simulink model "PMSM_Motor"  (R2013b)
settings: Solver=ode45  StartTime=0.0  StopTime=1  MaxStep=1e-4  RelTol=1e-3
values from neighbouring files (symbols this model uses):
  B = 0    [PMSM_Motorsimulator.m]
  f = 60    [PMSM_Motorsimulator.m]
  J = 0.0001584    [PMSM_Motorsimulator.m]
  L_d = 5.7e-3    (= 0.0057)    [PMSM_Motorsimulator.m]
  L_q = 12.5e-3    (= 0.0125)    [PMSM_Motorsimulator.m]
  Phi_pm = 175e-3    (= 0.175)    [PMSM_Motorsimulator.m]
  Rs = 1.2    [PMSM_Motorsimulator.m]
  T_Load = 10    [PMSM_Motorsimulator.m]
  U = 230    [PMSM_Motorsimulator.m]
  Zp = 2    [PMSM_Motorsimulator.m]
settings Model: Creator=ahakimi  LastModifiedBy=ahakimi

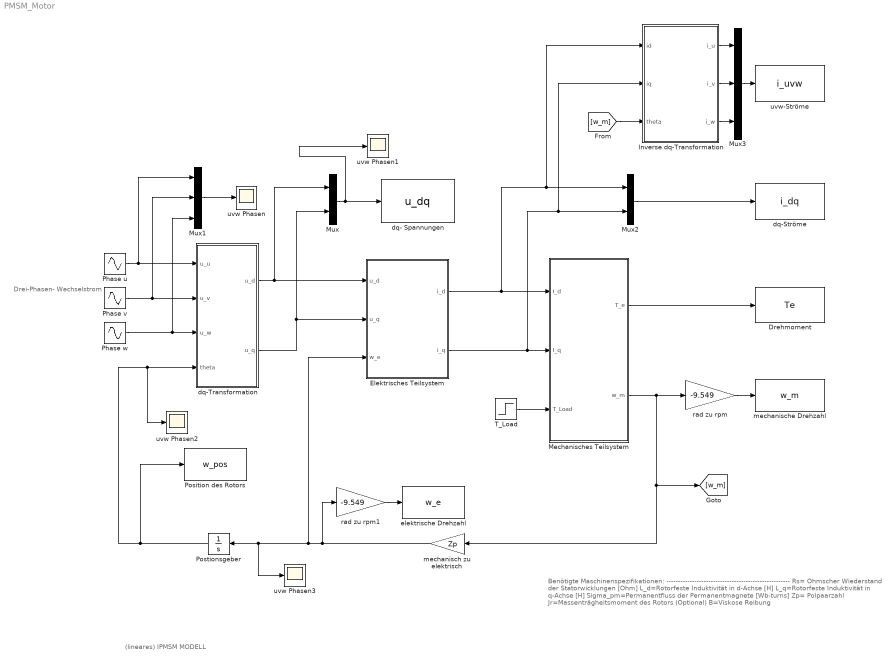
== system PMSM_Motor ==
  note: (lineares) IPMSM MODELL
  note: Drei-Phasen-
      | Wechselstrom
  note: Benötigte Maschinenspezifikationen:
      | -----------------------------------------------------
      | Rs= Ohmscher Wiederstand der Statorwicklungen [Ohm]
      | L_d=Rotorfeste Induktivität in d-Achse [H]
      | L_q=Rotorfeste Induktivität in q-Achse [H]
      | Sigma_pm=Permanentfluss der Permanentmagnete [Wb-turns]
      | Zp= Polpaarzahl
      | Jr=Massenträgheitsmoment des Rotors
      | (Optional) B=Viskose Reibung
  " mechanisch zu elektrisch " : Gain  Gain=Zp
  Drehmoment : ToWorkspace  VariableName=Te  SampleTime=-1  SaveFormat=Timeseries
  Elektrisches Teilsystem : Subsystem
  Inverse dq-Transformation : Subsystem
  Mechanisches Teilsystem : Subsystem
  Mux : Mux  Inputs=2
  Mux1 : Mux  Inputs=3
  Mux2 : Mux  Inputs=2
  Mux3 : Mux  Inputs=3
  Phase u : Sin  Amplitude=U  Frequency=2*pi*f  SampleTime=0
  Phase v : Sin  Amplitude=U  Frequency=2*pi*f  Phase=2*pi/3  SampleTime=0
  Phase w : Sin  Amplitude=U  Frequency=2*pi*f  Phase=-2*pi/3  SampleTime=0
  Position des Rotors : ToWorkspace  VariableName=w_pos  SampleTime=-1  SaveFormat=Timeseries
  Postionsgeber : Integrator
  T_Load : Step  Time=0.15  After=T_Load  SampleTime=0
  dq- Spannungen : ToWorkspace  VariableName=u_dq  SampleTime=-1  SaveFormat=Timeseries
  dq-Ströme : ToWorkspace  VariableName=i_dq  SampleTime=-1  SaveFormat=Timeseries
  dq-Transformation : Subsystem
  elektrische Drehzahl : ToWorkspace  VariableName=w_e  SampleTime=-1  SaveFormat=Timeseries
  mechanische Drehzahl : ToWorkspace  VariableName=w_m  SampleTime=-1  SaveFormat=Timeseries
  rad zu rpm : Gain  Gain=-9.549
  rad zu rpm1 : Gain  Gain=-9.549
  uvw Phasen{,1..3} (4 alike) : Scope
      uvw Phasen settings: YMin=-250  YMax=250  SaveName=ScopeData2
      uvw Phasen1 settings: YMin=-250  YMax=250
      uvw Phasen2 settings: YMin=-250  YMax=250
      uvw Phasen3 settings: YMin=-250  YMax=250  SaveName=ScopeData3
  uvw-Ströme : ToWorkspace  VariableName=i_uvw  SampleTime=-1  SaveFormat=Timeseries
  wires:
  Phase u/1 -> dq-Transformation/1(u_u), Mux1/1
  Phase v/1 -> dq-Transformation/2(u_v), Mux1/2
  Phase w/1 -> Mux1/3, dq-Transformation/3(u_w)
  Elektrisches Teilsystem/1(i_d) -> Inverse dq-Transformation/1(id), Mux2/1, Mechanisches Teilsystem/1(I_d)
  Mux1/1 -> uvw Phasen/1
  Mux/1 -> dq- Spannungen/1, uvw Phasen1/1
  Mechanisches Teilsystem/2(w_m) -> [w_m], " mechanisch zu elektrisch "/1, rad zu rpm/1
  rad zu rpm/1 -> mechanische Drehzahl/1
  Mechanisches Teilsystem/1(T_e) -> Drehmoment/1
  " mechanisch zu elektrisch "/1 -> rad zu rpm1/1, uvw Phasen3/1, Postionsgeber/1, Elektrisches Teilsystem/3(w_e)
  Postionsgeber/1 -> Position des Rotors/1, uvw Phasen2/1, dq-Transformation/4(theta)
  Mux2/1 -> dq-Ströme/1
  dq-Transformation/2(u_q) -> Mux/2, Elektrisches Teilsystem/2(u_q)
  dq-Transformation/1(u_d) -> Mux/1, Elektrisches Teilsystem/1(u_d)
  Elektrisches Teilsystem/2(i_q) -> Mux2/2, Inverse dq-Transformation/2(iq), Mechanisches Teilsystem/2(I_q)
  Inverse dq-Transformation/1(i_u) -> Mux3/1
  Inverse dq-Transformation/2(i_v) -> Mux3/2
  Inverse dq-Transformation/3(i_w) -> Mux3/3
  Mux3/1 -> uvw-Ströme/1
  rad zu rpm1/1 -> elektrische Drehzahl/1
  T_Load/1 -> Mechanisches Teilsystem/3(T_Load)
  [w_m] -> Inverse dq-Transformation/3(theta)

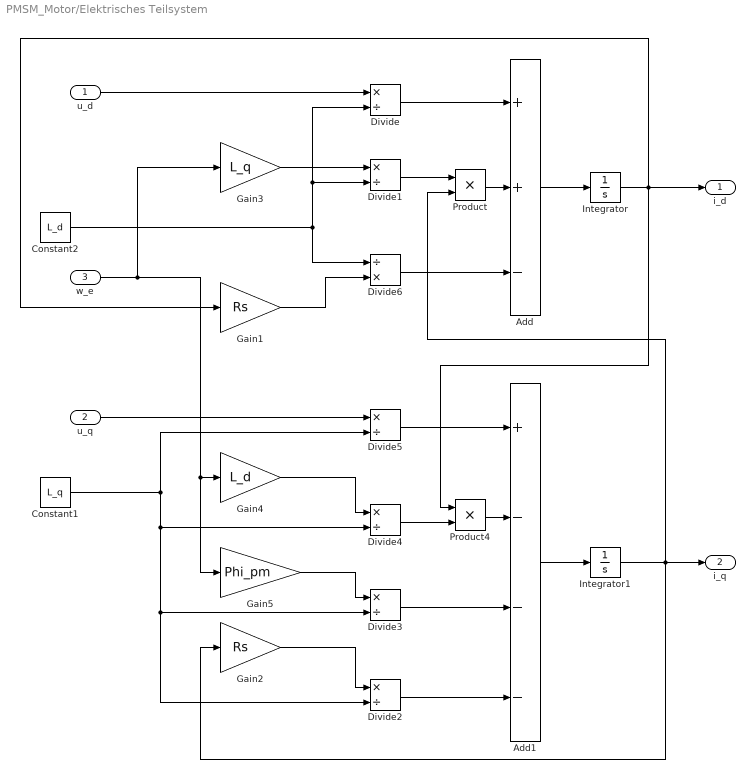
== system PMSM_Motor/Elektrisches Teilsystem ==
  u_d : Inport
  u_q : Inport  Port=2
  w_e : Inport  Port=3
  Add : Sum  Inputs=++-
  Add1 : Sum  Inputs=+---
  Constant1 : Constant  Value=L_q
  Constant2 : Constant  Value=L_d
  Divide{,1..5} (6 alike) : Product  Inputs=*/
  Divide6 : Product  Inputs=/*
  Gain1 : Gain  Gain=Rs
  Gain2 : Gain  Gain=Rs
  Gain3 : Gain  Gain=L_q
  Gain4 : Gain  Gain=L_d
  Gain5 : Gain  Gain=Phi_pm
  Integrator : Integrator
  Integrator1 : Integrator
  Product : Product
  Product4 : Product
  i_d : Outport
  i_q : Outport  Port=2
  wires:
  Divide1/1 -> Product/1
  Integrator1/1 -> i_q/1, Gain2/1, Product/2
  w_e/1 -> Gain3/1, Gain5/1, Gain4/1
  Constant2/1 -> Divide6/1, Divide/2, Divide1/2
  Divide/1 -> Add/1
  Divide3/1 -> Add1/3
  Gain1/1 -> Divide6/2
  Gain3/1 -> Divide1/1
  u_q/1 -> Divide5/1
  u_d/1 -> Divide/1
  Gain5/1 -> Divide3/1
  Divide5/1 -> Add1/1
  Product/1 -> Add/2
  Product4/1 -> Add1/2
  Constant1/1 -> Divide5/2, Divide2/2, Divide3/2, Divide4/2
  Gain4/1 -> Divide4/1
  Integrator/1 -> i_d/1, Gain1/1, Product4/1
  Divide4/1 -> Product4/2
  Gain2/1 -> Divide2/1
  Divide2/1 -> Add1/4
  Add/1 -> Integrator/1
  Add1/1 -> Integrator1/1
  Divide6/1 -> Add/3

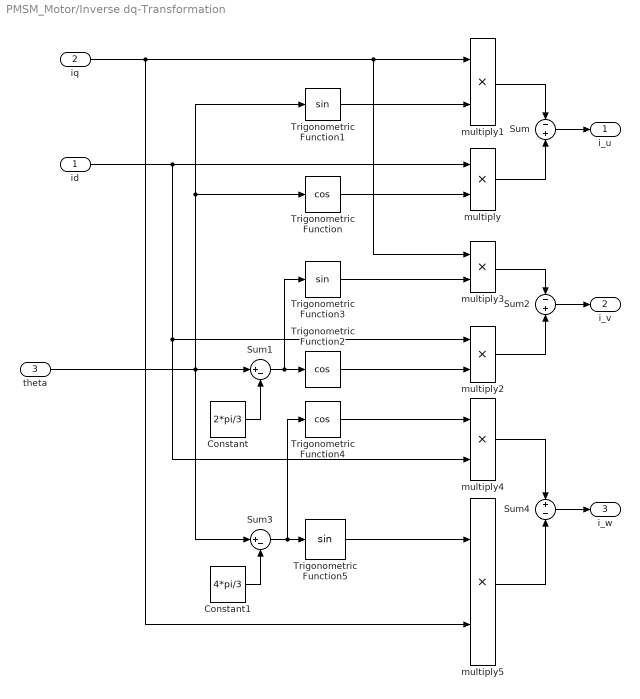
== system PMSM_Motor/Inverse dq-Transformation ==
  id : Inport
  iq : Inport  Port=2
  theta : Inport  Port=3
  Constant : Constant  Value=2*pi/3
  Constant1 : Constant  Value=4*pi/3
  Sum : Sum  Inputs=-|+
  Sum1 : Sum  Inputs=|+-
  Sum2 : Sum  Inputs=-|+
  Sum3 : Sum  Inputs=|+-
  Sum4 : Sum  Inputs=+|-
  Trigonometric Function : Trigonometry  Operator=cos
  Trigonometric Function1 : Trigonometry
  Trigonometric Function2 : Trigonometry  Operator=cos
  Trigonometric Function3 : Trigonometry
  Trigonometric Function4 : Trigonometry  Operator=cos
  Trigonometric Function5 : Trigonometry
  multiply{,1..5} (6 alike) : Product  Inputs=**
  i_u : Outport
  i_v : Outport  Port=2
  i_w : Outport  Port=3
  wires:
  Sum/1 -> i_u/1
  Sum2/1 -> i_v/1
  Trigonometric Function1/1 -> multiply1/2
  Trigonometric Function/1 -> multiply/2
  id/1 -> multiply4/2, multiply2/1, multiply/1
  multiply1/1 -> Sum/1
  multiply/1 -> Sum/2
  multiply3/1 -> Sum2/1
  Trigonometric Function3/1 -> multiply3/2
  Sum4/1 -> i_w/1
  Trigonometric Function4/1 -> multiply4/1
  Trigonometric Function5/1 -> multiply5/1
  multiply2/1 -> Sum2/2
  Sum3/1 -> Trigonometric Function5/1, Trigonometric Function4/1
  multiply5/1 -> Sum4/2
  Constant/1 -> Sum1/2
  Sum1/1 -> Trigonometric Function2/1, Trigonometric Function3/1
  Constant1/1 -> Sum3/2
  Trigonometric Function2/1 -> multiply2/2
  multiply4/1 -> Sum4/1
  theta/1 -> Sum3/1, Sum1/1, Trigonometric Function1/1, Trigonometric Function/1
  iq/1 -> multiply5/2, multiply3/1, multiply1/1

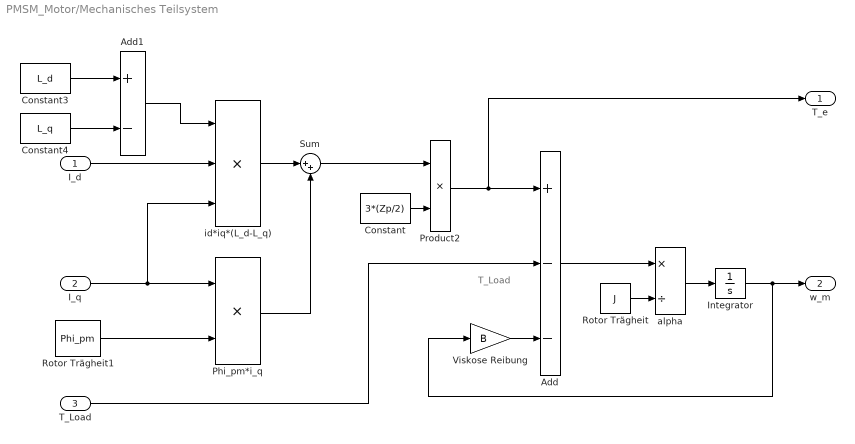
== system PMSM_Motor/Mechanisches Teilsystem ==
  note: T_Load
  I_d : Inport
  I_q : Inport  Port=2
  T_Load : Inport  Port=3
  Add : Sum  Inputs=+--
  Add1 : Sum  Inputs=+-
  Constant : Constant  Value=3*(Zp/2)
  Constant3 : Constant  Value=L_d
  Constant4 : Constant  Value=L_q
  Integrator : Integrator
  Phi_pm*i_q : Product
  Product2 : Product
  Rotor Trägheit : Constant  Value=J
  Rotor Trägheit1 : Constant  Value=Phi_pm
  Sum : Sum  Inputs=|++
  Viskose Reibung : Gain  Gain=B
  alpha : Product  Inputs=*/
  id*iq*(L_d-L_q) : Product  Inputs=3
  T_e : Outport
  w_m : Outport  Port=2
  wires:
  I_q/1 -> id*iq*(L_d-L_q)/3, Phi_pm*i_q/1
  alpha/1 -> Integrator/1
  Phi_pm*i_q/1 -> Sum/2
  Constant/1 -> Product2/2
  Add/1 -> alpha/1
  Rotor Trägheit/1 -> alpha/2
  Integrator/1 -> Viskose Reibung/1, w_m/1
  Viskose Reibung/1 -> Add/3
  Product2/1 -> Add/1, T_e/1
  Sum/1 -> Product2/1
  Constant3/1 -> Add1/1
  Constant4/1 -> Add1/2
  I_d/1 -> id*iq*(L_d-L_q)/2
  Add1/1 -> id*iq*(L_d-L_q)/1
  Rotor Trägheit1/1 -> Phi_pm*i_q/2
  id*iq*(L_d-L_q)/1 -> Sum/1
  T_Load/1 -> Add/2

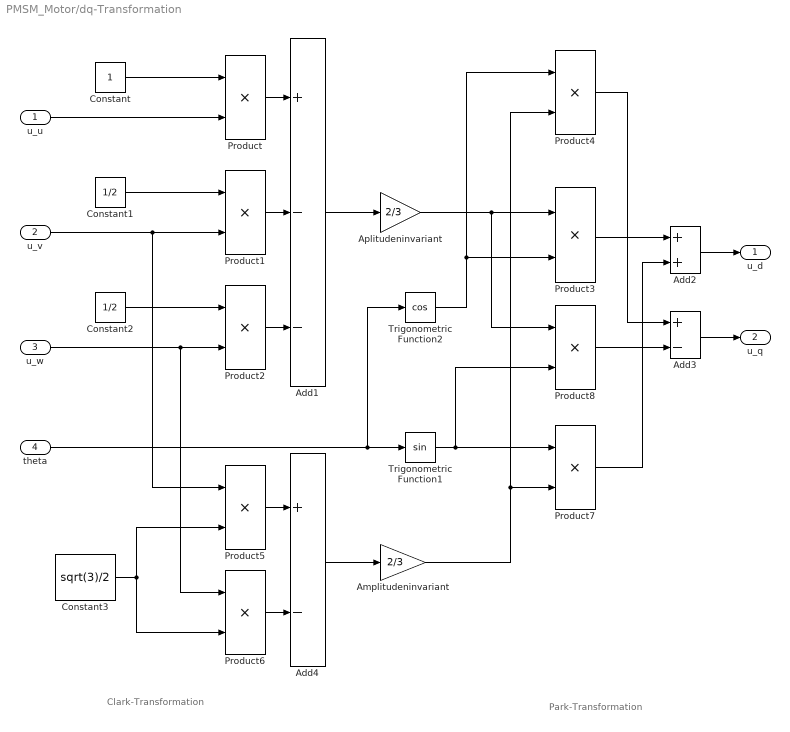
== system PMSM_Motor/dq-Transformation ==
  note: Park-Transformation
  note: Clark-Transformation
  u_u : Inport
  u_v : Inport  Port=2
  u_w : Inport  Port=3
  theta : Inport  Port=4
  Add1 : Sum  Inputs=+--
  Add2 : Sum
  Add3 : Sum  Inputs=+-
  Add4 : Sum  Inputs=+-
  Amplitudeninvariant : Gain  Gain=2/3
  Aplitudeninvariant : Gain  Gain=2/3
  Constant : Constant
  Constant1 : Constant  Value=1/2
  Constant2 : Constant  Value=1/2
  Constant3 : Constant  Value=sqrt(3)/2
  Product{,1..8} (9 alike) : Product
  Trigonometric Function1 : Trigonometry
  Trigonometric Function2 : Trigonometry  Operator=cos
  u_d : Outport
  u_q : Outport  Port=2
  wires:
  Add3/1 -> u_q/1
  Trigonometric Function1/1 -> Product8/2, Product7/1
  Add1/1 -> Aplitudeninvariant/1
  Constant3/1 -> Product5/2, Product6/2
  Add2/1 -> u_d/1
  Product8/1 -> Add3/2
  Trigonometric Function2/1 -> Product4/1, Product3/2
  u_u/1 -> Product/2
  Product2/1 -> Add1/3
  Product1/1 -> Add1/2
  Constant/1 -> Product/1
  Product5/1 -> Add4/1
  Constant1/1 -> Product1/1
  Product6/1 -> Add4/2
  Product3/1 -> Add2/1
  Add4/1 -> Amplitudeninvariant/1
  Product/1 -> Add1/1
  u_w/1 -> Product6/1, Product2/2
  Product7/1 -> Add2/2
  Product4/1 -> Add3/1
  Constant2/1 -> Product2/1
  u_v/1 -> Product1/2, Product5/1
  Aplitudeninvariant/1 -> Product3/1, Product8/1
  Amplitudeninvariant/1 -> Product4/2, Product7/2
  theta/1 -> Trigonometric Function2/1, Trigonometric Function1/1
